simulink model "Bicycle_Simulink"  (R2024a)
settings: Solver=VariableStepAuto  StartTime=0.0  StopTime=10.0  RelTol=1e-3
undefined symbols (not defined in the file or in its folder): sigbuilder_block, Transformador
settings Model: Creator=Vilson Wenis Belle  LastModifiedBy=wenis
settings SolverCC: AlgebraicLoopSolver=TrustRegion
settings DebuggingCC: UnconnectedInputMsg=warning  UnconnectedOutputMsg=warning  UnconnectedLineMsg=warning
settings ModelReferenceCC: EnableRefExpFcnMdlSchedulingChecks=on
settings RTWCC: GPUComputeCapability=3.5  DLArmComputeVersion=19.05

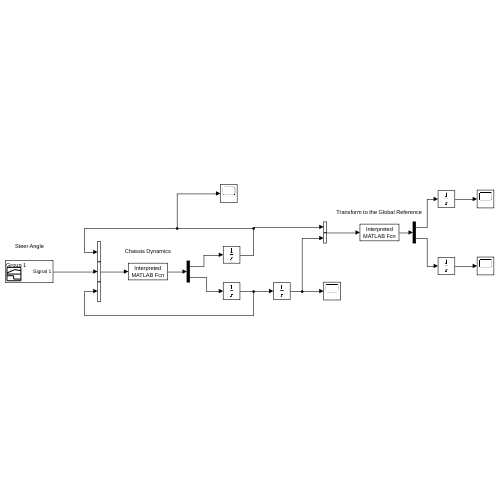
[thumbnail: Simulink's stored preview of the top-level diagram]
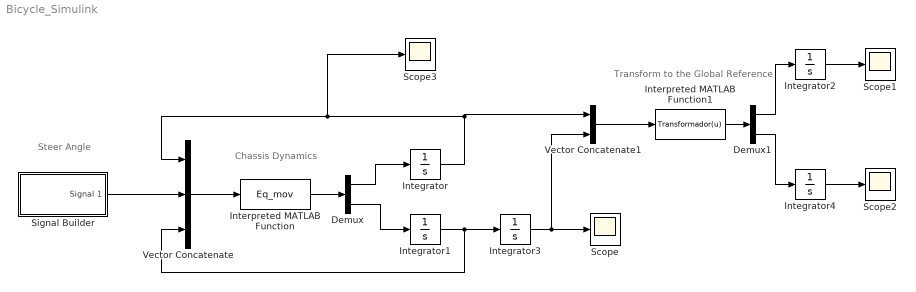
== system Bicycle_Simulink ==
  note: Transform to the Global Reference
  note: Chassis Dynamics
  note: Steer Angle
  Demux : Demux  Outputs=2
  Demux1 : Demux  Outputs=2
  Integrator{,1..4} (5 alike) : Integrator
  Interpreted MATLAB Function : MATLABFcn  MATLABFcn=Eq_mov  OutputDimensions=2
  Interpreted MATLAB Function1 : MATLABFcn  MATLABFcn=Transformador(u)  OutputDimensions=2
  Scope{,1..3} (4 alike) : Scope
  Signal Builder : Subsystem  Tag=STV Subsys  LoadFcn=sigbuilder_block('load');  StartFcn=sigbuilder_block('start');  StopFcn=sigbuilder_block('stop');  ClipboardFcn=sigbuilder_block('clipboard');  mask(Sigbuilder block){tuvar=[0:10]}
      mask help: Simulink:masks:SigbuilderBlock_MD
      mask init:
      | if ~strcmp(get_param(bdroot(gcbh),'SimulationStatus'),'stopped') tuvar = sigbuilder_block('maskInit'); end
      settings: CopyFcn=sigbuilder_block('copy');  DeleteFcn=sigbuilder_block('delete');  ModelCloseFcn=sigbuilder_block('modelClose');  PreSaveFcn=sigbuilder_block('preSave');  PauseFcn=sigbuilder_block('pause');  ContinueFcn=sigbuilder_block('continue');  NameChangeFcn=sigbuilder_block('namechange');  OpenFcn=sigbuilder_block('open',[437.25 153 550.5 359.25 ]);  CloseFcn=sigbuilder_block('close');
      mask Display: plot(0, 0, 100, 100,[2, 2, 32, 32, 2], [68, 8, 8, 68, 68],[32, 2], [38, 38], [32, 19, 2],[53, 60, 44], [32, 17, 17, 2],[16, 16, 31, 31]);txt = getActiveGroup(gcbh);text(2, 100, txt,'verticalAlignment', 'top');
  Vector Concatenate : Concatenate  NumInputs=3
  Vector Concatenate1 : Concatenate
  wires:
  Vector Concatenate/1 -> Interpreted MATLAB Function/1
  Interpreted MATLAB Function/1 -> Demux/1
  Signal Builder/1(Signal 1) -> Vector Concatenate/2
  Demux/1 -> Integrator/1
  Demux/2 -> Integrator1/1
  Integrator/1 -> Scope3/1, Vector Concatenate/1, Vector Concatenate1/1
  Integrator1/1 -> Integrator3/1, Vector Concatenate/3
  Integrator3/1 -> Vector Concatenate1/2, Scope/1
  Vector Concatenate1/1 -> Interpreted MATLAB Function1/1
  Interpreted MATLAB Function1/1 -> Demux1/1
  Demux1/2 -> Integrator4/1
  Demux1/1 -> Integrator2/1
  Integrator2/1 -> Scope1/1
  Integrator4/1 -> Scope2/1

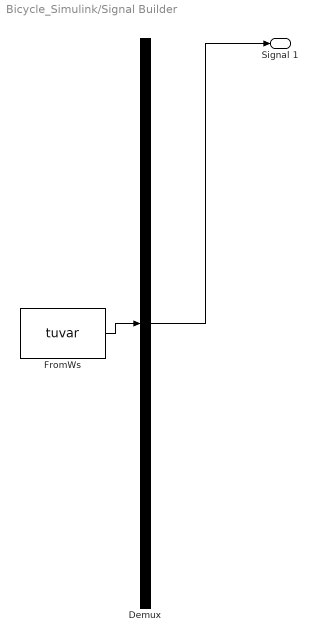
== system Bicycle_Simulink/Signal Builder ==
  Demux : Demux  Tag=STV Demux  Outputs=1
      settings: DisplayOption=none
  FromWs : FromWorkspace  Tag=STV FromWs  VariableName=tuvar
      SigBuilderData=|
      | common.afterFinalStr = 'Extrapolate'
      | common.sampleTime = 0
      | dataSet.timeRange = [0 10]
      | dataSet.name = 'Group 1'
      | sbobj.Groups.Name = 'Group 1'
      | sbobj.Groups.Signals.Name = 'Signal 1'
      | sbobj.Groups.Signals.XData = [0 0.10101010101 0.20202020202 0.30303030303 0.40404040404 0.505050505051 0.606060606061 0.707070707071 0.808080808081 0.909090909091 1.0101010101 1.11111111111 1.21212121212 1.31313131313 1.41414141414 1.51515151515 1.61616161616 1.71717171717 1.81818181818 1.91919191919 2.0202020202 2.12121212121 2.22222222222 2.32323232323 2.42424242424 2.52525252525 2.62626262626 2.72727272727 2.82828282828 2.92929292929 3.0303030303 3.13131313131 3.23232323232 3.33333333333 3.43434343434 3.53535353535 3.63636363636 3.73737373737 3.83838383838 3.93939393939 4.0404040404 4.14141414141 4.24242424242 4.34343434343 4.44444444444 4.54545454545 4.64646464646 4.74747474747 4.84848484848 4.94949494949 5.05050505051 5.15151515152 5.25252525253 5.35353535354 5.45454545455 5.55555555556 5.65656565657 5.75757575758 5.85858585859 5.9595959596 6.06060606061 6.16161616162 6.26262626263 6.36363636364 6.46464646465 6.56565656566 6.66666666667 6.76767676768 6.86868686869 6.9696969697 7.07070707071 7.17171717172 7.27272727273 7.37373737374 7.47474747475 7.57575757576 7.67676767677 7.77777777778 7.87878787879 7.9797979798 8.08080808081 8.18181818182 8.28282828283 8.38383838384 8.48484848485 8.58585858586 8.68686868687 8.78787878788 8.88888888889 8.9898989899 9.09090909091 9.19191919192 9.29292929293 9.39393939394 9.49494949495 9.59595959596 9.69696969697 9.79797979798 9.89898989899 10]
      | sbobj.Groups.Signals.YData = [0 0.0110695622253 0.0220945512304 0.0330305732759 0.0438335928607 0.0544601100378 0.0648673355732 0.0750133632428 0.084857338574 0.0943596233527 0.103481955232 0.112187601801 0.120441508493 0.128210439739 0.135463112796 0.142170323708 0.148305064905 0.153842633949 0.158760733004 0.163039558621 0.166661881479 0.169613115762 0.171881377892 0.173457534378 0.174335238594 0.174510956334 0.173983980046 0.172756431677 0.17083325413 0.168222191364 0.164933757206 0.16098119302 0.156380414388 0.15114994702 0.145310852162 0.13888664179 0.13190318393 0.124388598503 0.116373144092 0.107889096103 0.0989706168032 0.0896536177601 0.079975615241 0.0699755791463 0.0596937760918 0.0491716072695 0.0384514417395 0.0275764458248 0.0165904092958 0.00553756904395 -0.00553756904395 -0.0165904092958 -0.0275764458248 -0.0384514417395 -0.0491716072695 -0.0596937760918 -0.0699755791463 -0.079975615241 -0.0896536177601 -0.0989706168032 -0.107889096103 -0.116373144092 -0.124388598503 -0.13190318393 -0.13888664179 -0.145310852162 -0.15114994702 -0.156380414388 -0.16098119302 -0.164933757206 -0.168222191364 -0.17083325413 -0.172756431677 -0.173983980046 -0.174510956334 -0.174335238594 -0.173457534378 -0.171881377892 -0.169613115762 -0.166661881479 -0.163039558621 -0.158760733004 -0.153842633949 -0.148305064905 -0.142170323708 -0.135463112796 -0.128210439739 -0.120441508493 -0.112187601801 -0.103481955232 -0.0943596233527 -0.084857338574 -0.0750133632428 -0.0648673355732 -0.0544601100378 -0.0438335928607 -0.0330305732759 -0.0220945512304 -0.0110695622253 0]
  Signal 1 : Outport  Tag=STV Outport
  wires:
  Demux/1 -> Signal 1/1
  FromWs/1 -> Demux/1
